simulink model "labkit1-CANsend"  (R2021a)
settings: Solver=FixedStepDiscrete  StartTime=0.0  StopTime=inf  RelTol=1e-3  EnableMultiTasking=on
libraries: labkit_toolbox x4, canmsglib x1
settings Model: Creator=user  LastModifiedBy=user
settings SolverCC: PositivePriorityOrder=on  AutoInsertRateTranBlk=on
settings OptimizationCC: DefaultParameterBehavior=Inlined  EnhancedBackFolding=on  PassReuseOutputArgsAs=Individual arguments  ZeroExternalMemoryAtStartup=off  ZeroInternalMemoryAtStartup=off  OptimizeBlockOrder=speed  DifferentSizesBufferReuse=on  OptimizationCustomize=off  EfficientTunableParamExpr=on
settings DebuggingCC: ParameterTunabilityLossMsg=error
settings SFSimCC: MATLABDynamicMemAlloc=off
settings RTWCC: Description=Waijung 2 ESP32 target  SystemTargetFile=esp32.tlc  GenCodeOnly=on  MakeCommand=make_rtw TMF=1  GenerateMakefile=off  TemplateMakefile=ert_default_tmf  RetainRTWFile=on
settings CodeAppCC: ForceParamTrailComments=on  IgnoreCustomStorageClasses=off  OperatorAnnotations=on  SimulinkDataObjDesc=on  SFDataObjDesc=on  InsertBlockDesc=on
settings ERTTargetCC: TargetLangStandard=C99 (ISO)  UseToolchainInfoCompliant=off  InlinedParameterPlacement=NonHierarchical  ERTSrcFileBannerTemplate=esp32_code_template.cgt  ERTHdrFileBannerTemplate=esp32_code_template.cgt  ERTDataSrcFileTemplate=esp32_code_template.cgt  ERTDataHdrFileTemplate=esp32_code_template.cgt  ERTCustomFileTemplate=esp32_file_process.tlc

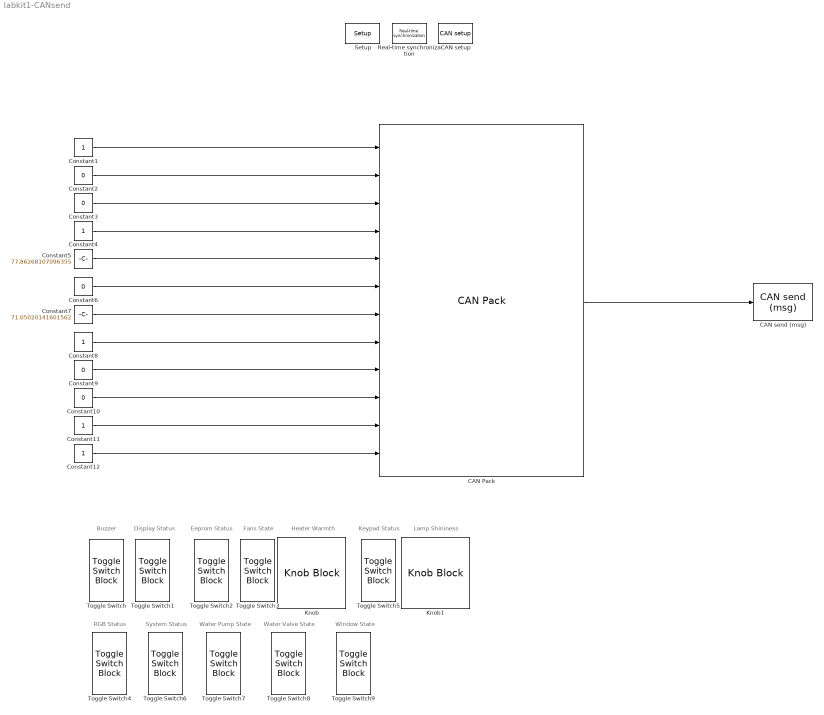
== system labkit1-CANsend ==
  note: Window State
  note: Water Valve State
  note: Water Pump State
  note: System Status
  note: RGB Status
  note: Lamp Shininess
  note: Keypad Status
  note: Heater Warmth
  note: Fans State
  note: Eeprom Status
  note: Display Status
  note: Buzzer
  CAN Pack : canmsglib/CAN Pack  CANdbFile=C:\Users\user\Desktop\greenhouse.dbc  MsgList=hmi  MsgName=hmi  MsgIDType=Standard (11-bit identifier)  MsgIdentifier=258  MsgLength=8  Remote=off  ApplyMinMax=off  BusOutput=on  SignalInfo={'buzzer_status','40','2','LE','unsigned','Standard','0','1','0','-Inf','Inf';'display_status','36','2','LE','unsigned','Standard','0','1','0','-Inf','Inf';'eeprom_status','44','2','LE','unsigned','Standard','0','1','0','-Inf','Inf';'fans_state','22','1','LE','unsigned','Standard','0','1','0','-Inf','Inf';'heater_warmness','8','7','LE','unsigned','Standard','0','1','0','0','100';'keypad_status','38','2','LE','unsigned','Standard','0','1','0','-Inf','Inf';'lamp_shininess','0','7','LE','unsigned','Standard','0','1','0','0','100';'rgb_status','42','2','LE','unsigned','Standard','0','1','0','-Inf','Inf';'system_status','46','2','LE','unsigned','Standard','0','1','0','-Inf','Inf';'water_pump_state','16','1','LE','unsigned','Standard','0','1','0','-Inf','Inf';'water_valve_state','18','1','LE','unsigned','Standard','0','1','0','-Inf','Inf';'window_state','20','1','LE','unsigned','Standard','0','1','0','-Inf','Inf'}
      settings: SourceProductBaseCode=ME,XP,VN  DataFormat=CANdb specified signals
  CAN send (msg) : labkit_toolbox/CAN send (msg)  frame_id=258  sample_time=1
      settings: SourceProductName=Lab kit toolbox
  CAN setup : labkit_toolbox/CAN setup  brp=10  tseg1=8  tseg2=7  sjw=1
      settings: SourceProductName=Lab kit toolbox
  Constant1 : Constant  VectorParams1D=off  OutDataTypeStr=uint8  SampleTime=0.1
  Constant{2..3,6,9..10} (5 alike) : Constant  Value=0
  Constant{4,8,11..12} (4 alike) : Constant
  Constant5 : Constant  Value=77.86268107096355
  Constant7 : Constant  Value=71.05020141601562
  Knob : KnobBlock
  Knob1 : KnobBlock
  Real-time synchronization : labkit_toolbox/Real-time synchronization  time_step=0.1
      settings: SourceProductName=Lab kit toolbox
  Setup : labkit_toolbox/Setup  port=COM4
      settings: SourceProductName=Lab kit toolbox
  Toggle Switch{,1..9} (10 alike) : ToggleSwitchBlock
      settings: Values={{'Off', 'On'}, [0 1]}
  wires:
  CAN Pack/1 -> CAN send (msg)/1
  Constant1/1 -> CAN Pack/1
  Constant2/1 -> CAN Pack/2
  Constant3/1 -> CAN Pack/3
  Constant4/1 -> CAN Pack/4
  Constant5/1 -> CAN Pack/5
  Constant6/1 -> CAN Pack/6
  Constant7/1 -> CAN Pack/7
  Constant8/1 -> CAN Pack/8
  Constant9/1 -> CAN Pack/9
  Constant10/1 -> CAN Pack/10
  Constant11/1 -> CAN Pack/11
  Constant12/1 -> CAN Pack/12
